simulink model "ammclib_gmclib_foc_F32_s32k11x"  (Simulink 9.0)
settings: Solver=FixedStepDiscrete  StartTime=0.0  StopTime=5  FixedStep=0.001  RelTol=1e-3  EnableMultiTasking=on
InitFcn:
  | mbd_s32k_consistency_checks(bdroot(gcs));
undefined symbols (not defined in the file): LQFP, thumb
libraries: ammclib_bam_s32k11x x22, mbd_s32k1xx_ec_toolbox x2, simulink x1
Description:
  | This model tests the AMMCLIB GMCLIB F32 blocks
  | 
  | Validation:
  | - Run the model in Simulation and check the results
  | - Open Freemaster (ammclib_gflib_foc_F32_s32k11x.pmp) and compare the HW results against the Simulated ones
CloseFcn:
  | clear all;
settings Model: Creator=NXP MBDT Team  LastModifiedBy=nxf35172
settings DataIOCC: ExternalInput=off  InitialState=off  LimitDataPoints=on  SaveOutput=off  SignalLogging=off  SaveTime=off
settings OptimizationCC: DefaultParameterBehavior=Inlined  PassReuseOutputArgsAs=Individual arguments  LifeSpan=auto
settings DebuggingCC: SolverPrmCheckMsg=warning  InheritedTsInSrcMsg=none  SingleTaskRateTransMsg=error  IntegerOverflowMsg=none  ParameterPrecisionLossMsg=none  ParameterTunabilityLossMsg=error  UnconnectedInputMsg=error  UnconnectedOutputMsg=error  UnconnectedLineMsg=error  AllowSymbolicDim=off  UnknownTsInhSupMsg=error  StateNameClashWarn=warning
settings HardwareCC: ProdLargestAtomicInteger=Long  ProdLargestAtomicFloat=Double  ProdIntDivRoundTo=Zero  ProdEndianess=LittleEndian  ProdHWDeviceType=ARM Compatible->ARM Cortex
settings SFSimCC: MATLABDynamicMemAlloc=off
settings RTWCC: SystemTargetFile=mbd_s32k.tlc  MakeCommand=mbd_s32k_make_rtw COPY_MDLREF_INCLUDES=0  TemplateMakefile=mbd_s32k.tmf  Description=Model Based Design Toolbox S32K14x Code Generation Target  GenerateReport=on  IncludeHyperlinkInReport=on  LaunchReport=on  GenerateTraceInfo=on  GenerateTraceReport=on  GenerateTraceReportSl=on  GenerateTraceReportSf=on  GenerateTraceReportEml=on
settings CodeAppCC: ForceParamTrailComments=on  IgnoreCustomStorageClasses=off  OperatorAnnotations=on  SimulinkDataObjDesc=on  SFDataObjDesc=on  InsertBlockDesc=on  StateflowObjectComments=off
settings STFCustomTargetCC: MultiwordLength=256  ModelReferenceCompliant=off  CombineOutputUpdateFcns=on  ERTCustomFileBanners=on  SupportContinuousTime=off  SupportNonInlinedSFcns=off  RemoveResetFunc=on  MATLABClassNameForMDSCustomization=Simulink.SoftwareTarget.ERTCustomization  GRTInterface=off  SystemTargetFile=mbd_s32k.tlc
settings ERTTargetCC: ModelReferenceCompliant=off  ParMdlRefBuildCompliant=off  CompOptLevelCompliant=off  ConcurrentExecutionCompliant=off  ModelStepFunctionPrototypeControlCompliant=off  CPPClassGenCompliant=off  UseToolchainInfoCompliant=off  InlinedParameterPlacement=NonHierarchical  ERTCustomFileTemplate=example_file_process.tlc

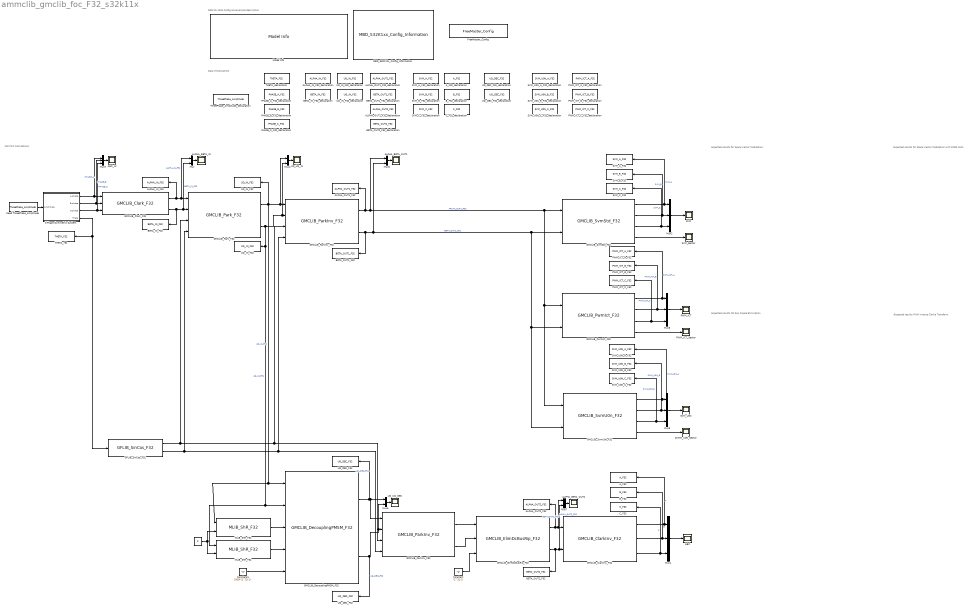
== system ammclib_gmclib_foc_F32_s32k11x ==
  note: Expected results DC Bus Ripple Elimination
  note: Expected results for Space Vector Modulation:
  note: S32K11x EVB Config and example description
  note: Data Initializations
  note: F32 FOC Calculations
  note: Expected results for Space Vector Modulation with O000 Nulls:
  note: Expected results PWM Inverse Clarke Transform
  " " : Constant  Value=2  OutDataTypeStr=Inherit: Inherit via back propagation
  " Read ThreePhase_Amplitude" : DataStoreRead  DataStoreName=ThreePhase_Amplitude
  3 Phase Symmetric System : Subsystem
  ABC : Scope
  ABC_IN : Scope
  ALPHA_BETA_IN : Scope
  ALPHA_BETA_OUT1 : Scope
  ALPHA_BETA_OUT2 : Scope
  ALPHA_IN_F32 : DataStoreWrite  DataStoreName=ALPHA_IN_F32
  ALPHA_IN_F32_declaration : DataStoreMemory  Priority=2  DataStoreName=ALPHA_IN_F32  ReadBeforeWriteMsg=warning  WriteAfterWriteMsg=warning  WriteAfterReadMsg=warning  ShowAdditionalParam=off  OutDataTypeStr=int32
  ALPHA_OUT1_F32 : DataStoreWrite  DataStoreName=ALPHA_OUT1_F32
  ALPHA_OUT1_F32_declaration : DataStoreMemory  Priority=2  DataStoreName=ALPHA_OUT1_F32  ReadBeforeWriteMsg=warning  WriteAfterWriteMsg=warning  WriteAfterReadMsg=warning  ShowAdditionalParam=off  OutDataTypeStr=int32
  ALPHA_OUT2_F32 : DataStoreWrite  DataStoreName=ALPHA_OUT2_F32
  ALPHA_OUT2_F32_declaration : DataStoreMemory  Priority=2  DataStoreName=ALPHA_OUT2_F32  ReadBeforeWriteMsg=warning  WriteAfterWriteMsg=warning  WriteAfterReadMsg=warning  ShowAdditionalParam=off  OutDataTypeStr=int32
  A_F32 : DataStoreWrite  DataStoreName=A_F32
  A_F32_declaration : DataStoreMemory  Priority=2  DataStoreName=A_F32  ReadBeforeWriteMsg=warning  WriteAfterWriteMsg=warning  WriteAfterReadMsg=warning  ShowAdditionalParam=off  OutDataTypeStr=int32
  BETA_IN_F32 : DataStoreWrite  DataStoreName=BETA_IN_F32
  BETA_IN_F32_declaration : DataStoreMemory  Priority=2  DataStoreName=BETA_IN_F32  ReadBeforeWriteMsg=warning  WriteAfterWriteMsg=warning  WriteAfterReadMsg=warning  ShowAdditionalParam=off  OutDataTypeStr=int32
  BETA_OUT1_F32 : DataStoreWrite  DataStoreName=BETA_OUT1_F32
  BETA_OUT1_F32_declaration : DataStoreMemory  Priority=2  DataStoreName=BETA_OUT1_F32  ReadBeforeWriteMsg=warning  WriteAfterWriteMsg=warning  WriteAfterReadMsg=warning  ShowAdditionalParam=off  OutDataTypeStr=int32
  BETA_OUT2_F32 : DataStoreWrite  DataStoreName=BETA_OUT2_F32
  BETA_OUT2_F32_declaration : DataStoreMemory  Priority=2  DataStoreName=BETA_OUT2_F32  ReadBeforeWriteMsg=warning  WriteAfterWriteMsg=warning  WriteAfterReadMsg=warning  ShowAdditionalParam=off  OutDataTypeStr=int32
  B_F32 : DataStoreWrite  DataStoreName=B_F32
  B_F32_declaration : DataStoreMemory  Priority=2  DataStoreName=B_F32  ReadBeforeWriteMsg=warning  WriteAfterWriteMsg=warning  WriteAfterReadMsg=warning  ShowAdditionalParam=off  OutDataTypeStr=int32
  C_F32 : DataStoreWrite  DataStoreName=C_F32
  C_F32_declaration : DataStoreMemory  Priority=2  DataStoreName=C_F32  ReadBeforeWriteMsg=warning  WriteAfterWriteMsg=warning  WriteAfterReadMsg=warning  ShowAdditionalParam=off  OutDataTypeStr=int32
  Constant : Constant  Value=(2^31-1)  OutDataTypeStr=Inherit: Inherit via back propagation
  Constant1 : Constant  Value=1000*(2^15-1)  OutDataTypeStr=Inherit: Inherit via back propagation
  FreeMaster_Config : mbd_s32k1xx_ec_toolbox/Utility Blocks/FreeMaster_Config  interface=LPUART0  baudrate=19200  rxd=PTB0: [LPUART0_RX | Receive]  txd=PTB1: [LPUART0_TX | Transmit]  mode=Short Interrupt  isr_prio=3  show_adv_opts=on  use_scope=on  max_scope_vars=8  use_recorder=on  max_rec_vars=8  rec_buff_size=1024  rec_timebase=0 seconds  comm_buffer_size_auto=on  comm_buffer_size=255  comm_rqueue_size_default=on  comm_rqueue_size=32
  GFLIB_SinCos_F32 : ammclib_bam_s32k11x/GFLIB/bam_f32/GFLIB_SinCos_F32
  GMCLIB_ClarkInv_F32 : ammclib_bam_s32k11x/GMCLIB/bam_f32/GMCLIB_ClarkInv_F32
  GMCLIB_Clark_F32 : ammclib_bam_s32k11x/GMCLIB/bam_f32/GMCLIB_Clark_F32
  GMCLIB_DecouplingPMSM_F32 : ammclib_bam_s32k11x/GMCLIB/bam_f32/GMCLIB_DecouplingPMSM_F32  f32Kd=0.625*(2^31-1)  s16KdShift=6  f32Kq=0.625*(2^31-1)  s16KqShift=5
  GMCLIB_ElimDcBusRip_F32 : ammclib_bam_s32k11x/GMCLIB/bam_f32/GMCLIB_ElimDcBusRip_F32  f32ModIndex=0.866025403784439*(2^31-1)
  GMCLIB_ParkInv_F32 : ammclib_bam_s32k11x/GMCLIB/bam_f32/GMCLIB_ParkInv_F32
  "GMCLIB_ParkInv_F32 " : ammclib_bam_s32k11x/GMCLIB/bam_f32/GMCLIB_ParkInv_F32
  GMCLIB_Park_F32 : ammclib_bam_s32k11x/GMCLIB/bam_f32/GMCLIB_Park_F32
  GMCLIB_PwmIct_F32 : ammclib_bam_s32k11x/GMCLIB/bam_f32/GMCLIB_PwmIct_F32
  GMCLIB_SvmStd_F32 : ammclib_bam_s32k11x/GMCLIB/bam_f32/GMCLIB_SvmStd_F32
  GMCLIB_SvmU0n_F32 : ammclib_bam_s32k11x/GMCLIB/bam_f32/GMCLIB_SvmU0n_F32
  MBD_S32K11x_Config_Information : mbd_s32k1xx_ec_toolbox/MBD_S32K1xx_Config_Information  mbdt_ver=0  disp_str=|  config_params=[]  mcu_target_name=S32K116  mcu_target_package=48-LQFP  mcu_target_sram_size=17KB  mcu_system_clock_freq=40  mcu_xtal_freq=External 40  mcu_steptick_timer=LPIT Channel 0  mcu_steptick_prio=3  ds_import_enable=on  target_compiler=GCC  target_memory=FLASH  gcc_target_compile_opts=-mcpu=cortex-m0plus -mthumb -O1 -g -gstrict-dwarf  gcc_target_assemble_opts=-mcpu=cortex-m0plus -mthumb -g  gcc_target_link_opts=-mcpu=cortex-m0plus -mthumb  gcc_target_default_lcf=on  gcc_target_user_lcf=S32K116_17_flash.ld  ghs_target_compile_opts=-mcpu=cortexm0plus -mthumb -fsoft -Ogeneral -Wundef -Wimplicit-int -Wshadow -Wtrigraphs --no_commons --gnu_asm -gnu99 -gdwarf-2 -G  ghs_target_assemble_opts=-mcpu=cortexm0plus -mthumb -fsoft --gnu_asm  ghs_target_link_opts=-mcpu=cortexm0plus -mthumb -fsoft  ghs_target_default_lcf=on  ghs_target_user_lcf=S32K116_17_flash.ld  iar_target_compile_opts=--thumb -Ol -e --debug --dlib_config normal  iar_target_assemble_opts=--thumb  iar_target_link_opts=--no_exceptions --vfe --inline  iar_target_default_lcf=on  iar_target_user_lcf=S32K116_17_flash.icf  pil_download_enable=off  rbl_download_enable=on  rbl_start_delay=5000  rbl_download_interface=OpenSDA  rbl_restart_request=off  rbl_com_port=Custom  rbl_com_port_custom=COM1  pil_download_rate=57600  pil_opensda_drive=Custom  pil_opensda_drive_custom=D  pil_uart_instance=0  pil_uart_rx=PTA2: [LPUART0_RX | Receive]  pil_uart_tx=PTA3: [LPUART0_TX | Transmit]  FTM_PWM_PcrCheckEnDis=on  FTM_Input_Edge_Inputs_PcrCheckEnDis=on  FTM_Dual_Edge_Inputs_PcrCheckEnDis=on  FTM_Quadrature_Inputs_PcrCheckEnDis=on  FTM_Hall_Sensor_Inputs_PcrCheckEnDis=on  LPTMR_PcrCheckEnDis=on  PIT_PcrCheckEnDis=on  RTC_PcrCheckEnDis=on  FlexCAN_PcrCheckEnDis=on  LIN_PcrCheckEnDis=on  FlexIO_PcrCheckEnDis=on  LPI2C_PcrCheckEnDis=on  LPSPI_PcrCheckEnDis=on  LPUART_PcrCheckEnDis=on  CMP_PcrCheckEnDis=on  GPIO_OutputPcrCheckEnDis=on  GPIO_InputPcrCheckEnDis=on  SBC_PcrCheckEnDis=on  AMMCLIB_PcrCheckEnDis=on  FM_PcrCheckEnDis=on  Profile_PcrCheckEnDis=on  ConfigParams_PcrCheckEnDis=on  ModelRef_PcrCheckEnDis=on  PDB0_PcrCheckEnDis=on  CSEc_PcrCheckEnDis=on  eDMA_PcrCheckEnDis=on  ADC_PcrCheckEnDis=on  WDOG_PcrCheckEnDis=on
      | Target : S32K144-64KB_SRAM
      | Package : 100-pin
      | System clock : 80 MHz
      | XTAL clock : External 8 MHz
      | Compiler : IAR
      | Target Type : FLASH
      | Download Code after build : off
      | Step Tick Interrupt Priority : 15
  MLIB_ShR_F32 : ammclib_bam_s32k11x/MLIB/bam_f32/MLIB_ShR_F32
  "MLIB_ShR_F32 " : ammclib_bam_s32k11x/MLIB/bam_f32/MLIB_ShR_F32
  Model Info : simulink/Model-Wide Utilities/Model Info  Frame=off  DisplayStringWithTags=|  HorizontalTextAlignment=Left  LeftAlignmentValue=0.02
      | Model Name: %<ModelName>
      | 
      | Description: %<Description>
  Mux{,4..7} (5 alike) : Mux  Inputs=2
  Mux{1..3,8..9} (5 alike) : Mux  Inputs=3
  PHASE_A_F32_declaration : DataStoreMemory  Priority=2  DataStoreName=PHASE_A_F32  ReadBeforeWriteMsg=warning  WriteAfterWriteMsg=warning  WriteAfterReadMsg=warning  ShowAdditionalParam=off  OutDataTypeStr=int32
  PHASE_B_F32_declaration : DataStoreMemory  Priority=2  DataStoreName=PHASE_B_F32  ReadBeforeWriteMsg=warning  WriteAfterWriteMsg=warning  WriteAfterReadMsg=warning  ShowAdditionalParam=off  OutDataTypeStr=int32
  PHASE_C_F32_declaration : DataStoreMemory  Priority=2  DataStoreName=PHASE_C_F32  ReadBeforeWriteMsg=warning  WriteAfterWriteMsg=warning  WriteAfterReadMsg=warning  ShowAdditionalParam=off  OutDataTypeStr=int32
  PWM_ICT : Scope
  PWM_ICT_A_F32 : DataStoreWrite  DataStoreName=PWM_ICT_A_F32
  PWM_ICT_A_F32_declaration : DataStoreMemory  Priority=2  DataStoreName=PWM_ICT_A_F32  ReadBeforeWriteMsg=warning  WriteAfterWriteMsg=warning  WriteAfterReadMsg=warning  ShowAdditionalParam=off  OutDataTypeStr=int32
  PWM_ICT_B_F32 : DataStoreWrite  DataStoreName=PWM_ICT_B_F32
  PWM_ICT_B_F32_declaration : DataStoreMemory  Priority=2  DataStoreName=PWM_ICT_B_F32  ReadBeforeWriteMsg=warning  WriteAfterWriteMsg=warning  WriteAfterReadMsg=warning  ShowAdditionalParam=off  OutDataTypeStr=int32
  PWM_ICT_C_F32 : DataStoreWrite  DataStoreName=PWM_ICT_C_F32
  PWM_ICT_C_F32_declaration : DataStoreMemory  Priority=2  DataStoreName=PWM_ICT_C_F32  ReadBeforeWriteMsg=warning  WriteAfterWriteMsg=warning  WriteAfterReadMsg=warning  ShowAdditionalParam=off  OutDataTypeStr=int32
  PWM_ICT_Sector : Scope
  SVM : Scope
  SVMM_U0N_Sector : Scope
  SVM_A_F32 : DataStoreWrite  DataStoreName=SVM_A_F32
  SVM_A_F32_declaration : DataStoreMemory  Priority=2  DataStoreName=SVM_A_F32  ReadBeforeWriteMsg=warning  WriteAfterWriteMsg=warning  WriteAfterReadMsg=warning  ShowAdditionalParam=off  OutDataTypeStr=int32
  SVM_B_F32 : DataStoreWrite  DataStoreName=SVM_B_F32
  SVM_B_F32_declaration : DataStoreMemory  Priority=2  DataStoreName=SVM_B_F32  ReadBeforeWriteMsg=warning  WriteAfterWriteMsg=warning  WriteAfterReadMsg=warning  ShowAdditionalParam=off  OutDataTypeStr=int32
  SVM_C_F32 : DataStoreWrite  DataStoreName=SVM_C_F32
  SVM_C_F32_declaration : DataStoreMemory  Priority=2  DataStoreName=SVM_C_F32  ReadBeforeWriteMsg=warning  WriteAfterWriteMsg=warning  WriteAfterReadMsg=warning  ShowAdditionalParam=off  OutDataTypeStr=int32
  SVM_Sector : Scope
  SVM_U0N : Scope
  SVM_U0N_A_F32 : DataStoreWrite  DataStoreName=SVM_U0N_A_F32
  SVM_U0N_A_F32_declaration : DataStoreMemory  Priority=2  DataStoreName=SVM_U0N_A_F32  ReadBeforeWriteMsg=warning  WriteAfterWriteMsg=warning  WriteAfterReadMsg=warning  ShowAdditionalParam=off  OutDataTypeStr=int32
  SVM_U0N_B_F32 : DataStoreWrite  DataStoreName=SVM_U0N_B_F32
  SVM_U0N_B_F32_declaration : DataStoreMemory  Priority=2  DataStoreName=SVM_U0N_B_F32  ReadBeforeWriteMsg=warning  WriteAfterWriteMsg=warning  WriteAfterReadMsg=warning  ShowAdditionalParam=off  OutDataTypeStr=int32
  SVM_U0N_C_F32 : DataStoreWrite  DataStoreName=SVM_U0N_C_F32
  SVM_U0N_C_F32_declaration : DataStoreMemory  Priority=2  DataStoreName=SVM_U0N_C_F32  ReadBeforeWriteMsg=warning  WriteAfterWriteMsg=warning  WriteAfterReadMsg=warning  ShowAdditionalParam=off  OutDataTypeStr=int32
  THETA_declaration : DataStoreMemory  Priority=2  DataStoreName=THETA_F32  ReadBeforeWriteMsg=warning  WriteAfterWriteMsg=warning  WriteAfterReadMsg=warning  ShowAdditionalParam=off  OutDataTypeStr=int32
  THETA_res : DataStoreWrite  DataStoreName=THETA_F32
  ThreePhase_Amplitude_declaration : DataStoreMemory  Priority=1  DataStoreName=ThreePhase_Amplitude  WriteAfterWriteMsg=warning  WriteAfterReadMsg=warning  InitialValue=0.61*(2^31-1)  ShowAdditionalParam=off  OutMin=-(2^31-1)  OutMax=(2^31-1)  OutDataTypeStr=int32
  UD_DEC_F32 : DataStoreWrite  DataStoreName=UD_DEC_F32
  UD_DEC_F32_declaration : DataStoreMemory  Priority=2  DataStoreName=UD_DEC_F32  ReadBeforeWriteMsg=warning  WriteAfterWriteMsg=warning  WriteAfterReadMsg=warning  ShowAdditionalParam=off  OutDataTypeStr=int32
  UD_IN_F32 : DataStoreWrite  DataStoreName=UD_IN_F32
  UD_IN_F32_declaration : DataStoreMemory  Priority=2  DataStoreName=UD_IN_F32  ReadBeforeWriteMsg=warning  WriteAfterWriteMsg=warning  WriteAfterReadMsg=warning  ShowAdditionalParam=off  OutDataTypeStr=int32
  UD_UQ_DEC : Scope
  UD_UQ_IN : Scope
  UQ_DEC_F32 : DataStoreWrite  DataStoreName=UQ_DEC_F32
  UQ_DEC_F32_declaration : DataStoreMemory  Priority=2  DataStoreName=UQ_DEC_F32  ReadBeforeWriteMsg=warning  WriteAfterWriteMsg=warning  WriteAfterReadMsg=warning  ShowAdditionalParam=off  OutDataTypeStr=int32
  UQ_IN_F32 : DataStoreWrite  DataStoreName=UQ_IN_F32
  UQ_IN_F32_declaration : DataStoreMemory  Priority=2  DataStoreName=UQ_IN_F32  ReadBeforeWriteMsg=warning  WriteAfterWriteMsg=warning  WriteAfterReadMsg=warning  ShowAdditionalParam=off  OutDataTypeStr=int32
  wires:
  3 Phase Symmetric System/4(Theta) -> GFLIB_SinCos_F32/1, THETA_res/1
  " Read ThreePhase_Amplitude"/1 -> 3 Phase Symmetric System/1("Amplitude ")
  3 Phase Symmetric System/2(B-phase) -> Mux3/2, GMCLIB_Clark_F32/2  "PHASE_B"
  3 Phase Symmetric System/1(A-phase) -> GMCLIB_Clark_F32/1, Mux3/1  "PHASE_A"
  3 Phase Symmetric System/3(C-phase) -> Mux3/3, GMCLIB_Clark_F32/3  "PHASE_C"
  GMCLIB_Clark_F32/1 -> ALPHA_IN_F32/1, Mux/1, GMCLIB_Park_F32/1  "ALPHA_IN_F32"
  GMCLIB_Clark_F32/2 -> BETA_IN_F32/1, Mux/2, GMCLIB_Park_F32/2  "BETA_IN_F32"
  GFLIB_SinCos_F32/1 -> GMCLIB_Park_F32/3, GMCLIB_ParkInv_F32/3, "GMCLIB_ParkInv_F32 "/3
  GFLIB_SinCos_F32/2 -> GMCLIB_Park_F32/4, GMCLIB_ParkInv_F32/4, "GMCLIB_ParkInv_F32 "/4
  GMCLIB_Park_F32/1 -> UD_IN_F32/1, Mux4/1, GMCLIB_ParkInv_F32/1, MLIB_ShR_F32/1, GMCLIB_DecouplingPMSM_F32/1  "UD_IN_F32"
  GMCLIB_Park_F32/2 -> Mux4/2, GMCLIB_ParkInv_F32/2, UQ_IN_F32/1, "MLIB_ShR_F32 "/1, GMCLIB_DecouplingPMSM_F32/2  "UQ_IN_F32"
  GMCLIB_ParkInv_F32/1 -> ALPHA_OUT1_F32/1, Mux6/1, GMCLIB_SvmU0n_F32/1, GMCLIB_PwmIct_F32/1, GMCLIB_SvmStd_F32/1  "APLHA_OUT1_F32"
  GMCLIB_ParkInv_F32/2 -> BETA_OUT1_F32/1, Mux6/2, GMCLIB_SvmU0n_F32/2, GMCLIB_PwmIct_F32/2, GMCLIB_SvmStd_F32/2  "BETA_OUT1_F32"
  GMCLIB_ElimDcBusRip_F32/1 -> ALPHA_OUT2_F32/1, Mux7/1, GMCLIB_ClarkInv_F32/1  "ALPHA_OUT2_F32"
  GMCLIB_ElimDcBusRip_F32/2 -> BETA_OUT2_F32/1, Mux7/2, GMCLIB_ClarkInv_F32/2  "BETA_OUT2_F32"
  Constant/1 -> GMCLIB_ElimDcBusRip_F32/3
  Mux2/1 -> SVM/1
  GMCLIB_SvmStd_F32/1 -> SVM_A_F32/1, Mux2/1  "SVM_A"
  GMCLIB_SvmStd_F32/2 -> SVM_B_F32/1, Mux2/2  "SVM_B"
  GMCLIB_SvmStd_F32/3 -> SVM_C_F32/1, Mux2/3  "SVM_C"
  GMCLIB_SvmStd_F32/4 -> SVM_Sector/1
  Constant1/1 -> GMCLIB_DecouplingPMSM_F32/5
  MLIB_ShR_F32/1 -> GMCLIB_DecouplingPMSM_F32/3
  "MLIB_ShR_F32 "/1 -> GMCLIB_DecouplingPMSM_F32/4
  " "/1 -> MLIB_ShR_F32/2, "MLIB_ShR_F32 "/2
  GMCLIB_DecouplingPMSM_F32/1 -> Mux5/1, "GMCLIB_ParkInv_F32 "/1, UD_DEC_F32/1  "UD_DEC_F32"
  GMCLIB_DecouplingPMSM_F32/2 -> UQ_DEC_F32/1, Mux5/2, "GMCLIB_ParkInv_F32 "/2  "UQ_DEC_F32"
  "GMCLIB_ParkInv_F32 "/1 -> GMCLIB_ElimDcBusRip_F32/1
  "GMCLIB_ParkInv_F32 "/2 -> GMCLIB_ElimDcBusRip_F32/2
  Mux1/1 -> ABC/1
  GMCLIB_ClarkInv_F32/2 -> B_F32/1, Mux1/2  "B"
  GMCLIB_ClarkInv_F32/3 -> C_F32/1, Mux1/3  "C"
  GMCLIB_ClarkInv_F32/1 -> A_F32/1, Mux1/1  "A"
  Mux/1 -> ALPHA_BETA_IN/1
  Mux3/1 -> ABC_IN/1
  Mux4/1 -> UD_UQ_IN/1
  Mux5/1 -> UD_UQ_DEC/1
  Mux6/1 -> ALPHA_BETA_OUT1/1
  Mux7/1 -> ALPHA_BETA_OUT2/1
  GMCLIB_PwmIct_F32/4 -> PWM_ICT_Sector/1
  GMCLIB_PwmIct_F32/3 -> PWM_ICT_C_F32/1, Mux8/3  "PWM_ICT_C"
  GMCLIB_PwmIct_F32/2 -> PWM_ICT_B_F32/1, Mux8/2  "PWM_ICT_B"
  GMCLIB_PwmIct_F32/1 -> PWM_ICT_A_F32/1, Mux8/1  "PWM_ICT_A"
  Mux8/1 -> PWM_ICT/1
  Mux9/1 -> SVM_U0N/1
  GMCLIB_SvmU0n_F32/1 -> SVM_U0N_A_F32/1, Mux9/1  "SVM_U0N_A"
  GMCLIB_SvmU0n_F32/2 -> SVM_U0N_B_F32/1, Mux9/2  "SWM_U0N_B"
  GMCLIB_SvmU0n_F32/3 -> SVM_U0N_C_F32/1, Mux9/3  "SVM_U0N_C"
  GMCLIB_SvmU0n_F32/4 -> SVMM_U0N_Sector/1

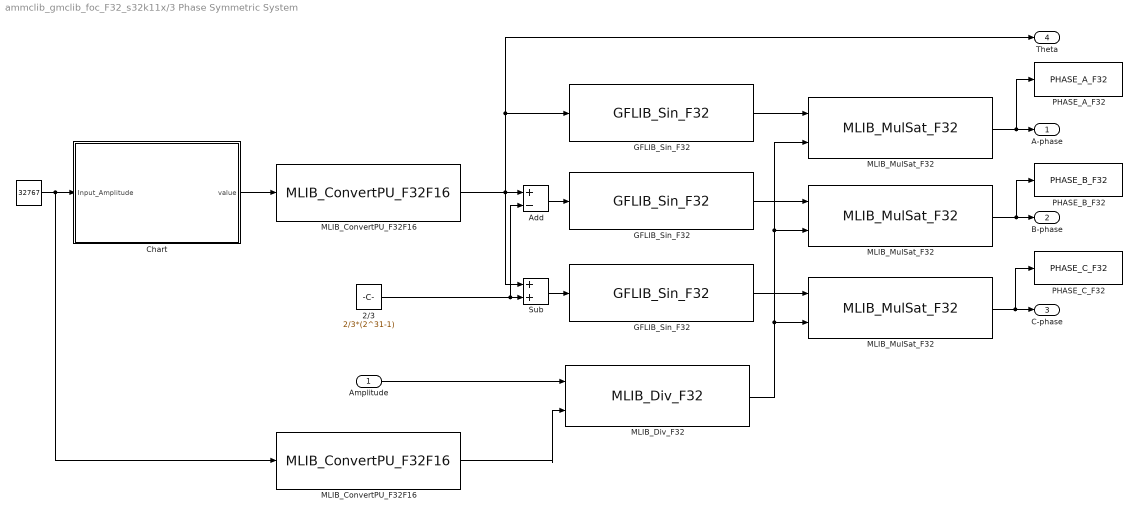
== system ammclib_gmclib_foc_F32_s32k11x/3 Phase Symmetric System ==
  "Amplitude " : Inport
  " " : Constant  Value=32767  OutDataTypeStr=int16
  2/3 : Constant  Value=2/3*(2^31-1)  OutDataTypeStr=int32
  Add : Sum  Inputs=+-
  Chart : Stateflow chart  TreatAsAtomicUnit=on
  GFLIB_Sin_F32 : ammclib_bam_s32k11x/GFLIB/bam_f32/GFLIB_Sin_F32
  "GFLIB_Sin_F32 " : ammclib_bam_s32k11x/GFLIB/bam_f32/GFLIB_Sin_F32
  "GFLIB_Sin_F32  " : ammclib_bam_s32k11x/GFLIB/bam_f32/GFLIB_Sin_F32
  MLIB_ConvertPU_F32F16 : ammclib_bam_s32k11x/MLIB/bam_f32/MLIB_ConvertPU_F32F16
  "MLIB_ConvertPU_F32F16    " : ammclib_bam_s32k11x/MLIB/bam_f32/MLIB_ConvertPU_F32F16
  MLIB_Div_F32 : ammclib_bam_s32k11x/MLIB/bam_f32/MLIB_Div_F32
  MLIB_MulSat_F32 : ammclib_bam_s32k11x/MLIB/bam_f32/MLIB_MulSat_F32
  "MLIB_MulSat_F32 " : ammclib_bam_s32k11x/MLIB/bam_f32/MLIB_MulSat_F32
  "MLIB_MulSat_F32  " : ammclib_bam_s32k11x/MLIB/bam_f32/MLIB_MulSat_F32
  PHASE_A_F32 : DataStoreWrite  DataStoreName=PHASE_A_F32
  PHASE_B_F32 : DataStoreWrite  DataStoreName=PHASE_B_F32
  PHASE_C_F32 : DataStoreWrite  DataStoreName=PHASE_C_F32
  Sub : Sum
  A-phase : Outport
  B-phase : Outport  Port=2
  C-phase : Outport  Port=3
  Theta : Outport  Port=4
  wires:
  Chart/1(value) -> MLIB_ConvertPU_F32F16/1
  " "/1 -> Chart/1(Input_Amplitude), "MLIB_ConvertPU_F32F16    "/1
  Sub/1 -> "GFLIB_Sin_F32  "/1
  Add/1 -> "GFLIB_Sin_F32 "/1
  MLIB_Div_F32/1 -> "MLIB_MulSat_F32  "/2, "MLIB_MulSat_F32 "/2, MLIB_MulSat_F32/2
  GFLIB_Sin_F32/1 -> MLIB_MulSat_F32/1
  "GFLIB_Sin_F32 "/1 -> "MLIB_MulSat_F32 "/1
  "GFLIB_Sin_F32  "/1 -> "MLIB_MulSat_F32  "/1
  MLIB_MulSat_F32/1 -> PHASE_A_F32/1, A-phase/1
  "MLIB_MulSat_F32 "/1 -> PHASE_B_F32/1, B-phase/1
  "MLIB_MulSat_F32  "/1 -> PHASE_C_F32/1, C-phase/1
  MLIB_ConvertPU_F32F16/1 -> Theta/1, GFLIB_Sin_F32/1, Sub/1, Add/1
  2/3/1 -> Add/2, Sub/2
  "Amplitude "/1 -> MLIB_Div_F32/1
  "MLIB_ConvertPU_F32F16    "/1 -> MLIB_Div_F32/2

== stateflow chart 3 Phase Symmetric System/Chart ==
  settings: executeAtInitialization=1
  state A
    du:
    cntr=cntr+25;
    value=cntr;
    ex:
    cntr = -Input_Amplitude;
  (default) -> A : {cntr=0;}
  A -> A : [cntr >= Input_Amplitude]
  data: cntr local int16 =0; value output int16; Input_Amplitude input int16
